simulink model "motor_control"  (R2021b)
settings: Solver=FixedStepAuto  StartTime=0.0  StopTime=inf  RelTol=1e-3  EnableMultiTasking=on
libraries: arduinomotorcarrierlib x4, simulink x2, arduinolib x1
settings Model: ExtModeTrigDuration=2  Creator=bkhusain  LastModifiedBy=cirie
settings SolverCC: AlgebraicLoopSolver=TrustRegion
settings OptimizationCC: EnhancedBackFolding=on  PassReuseOutputArgsAs=Individual arguments  ZeroExternalMemoryAtStartup=off  ZeroInternalMemoryAtStartup=off  MaxStackSize=64  OptimizeBlockOrder=speed  DifferentSizesBufferReuse=on  OptimizationCustomize=off  EfficientTunableParamExpr=on
settings DebuggingCC: ParameterTunabilityLossMsg=error  SFMachineParentedDataDiag=warning
settings HardwareCC: ProdBitPerPointer=32  ProdBitPerSizeT=32  ProdBitPerPtrDiffT=32  ProdLargestAtomicInteger=Long  ProdLargestAtomicFloat=Double  ProdWordSize=32  ProdHWDeviceType=ARM Compatible->ARM Cortex
settings SFSimCC: MATLABDynamicMemAlloc=off
settings RTWCC: Description=Embedded Coder  SystemTargetFile=ert.tlc  HardwareBoard=Arduino MKR WiFi 1010  TemplateMakefile=ert_default_tmf  Toolchain=Arduino ARM  BuildConfiguration=Faster Runs
settings CodeAppCC: ForceParamTrailComments=on  IgnoreCustomStorageClasses=off  OperatorAnnotations=on  SimulinkDataObjDesc=on  SFDataObjDesc=on  InsertBlockDesc=on
settings ERTTargetCC: SupportContinuousTime=on  SupportVariableSizeSignals=on  ExtModeTransport=3  ExtModeStaticAlloc=on  ExtModeStaticAllocSize=8192  ExtModeMexFile=ext_xcp  ExtModeIntrfLevel=Level2 - Open

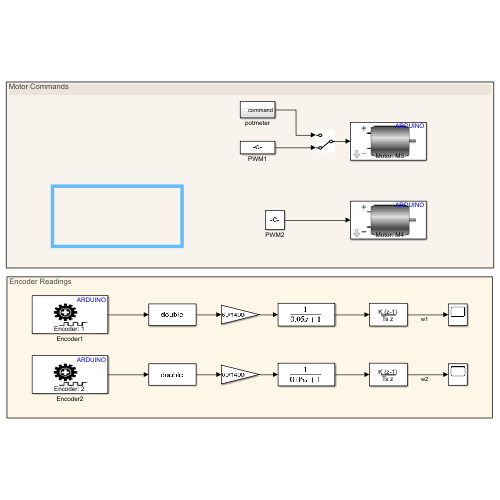
[thumbnail: Simulink's stored preview of the top-level diagram]
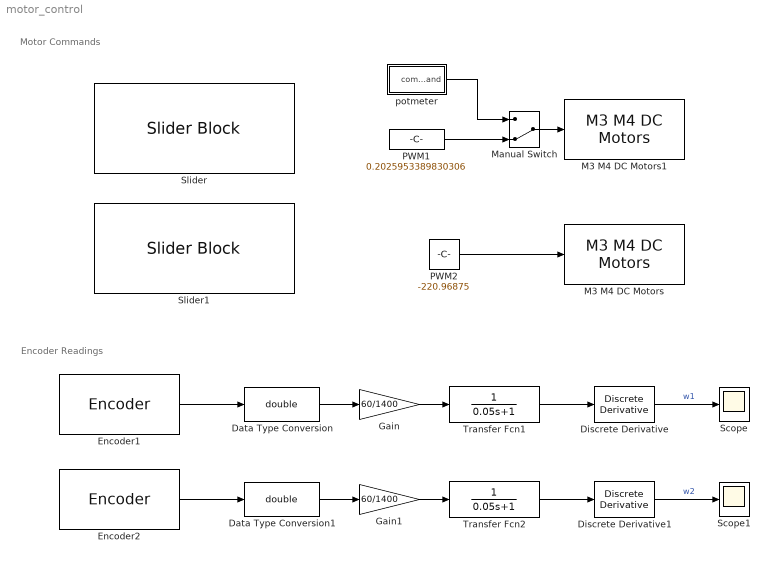
== system motor_control ==
  note: Encoder Readings
  note: Motor Commands
  Data Type Conversion : DataTypeConversion  OutDataTypeStr=double
  Data Type Conversion1 : DataTypeConversion  OutDataTypeStr=double
  Discrete Derivative : simulink/Discrete/Discrete Derivative  gainval=1.0  ICPrevScaledInput=0.0  OutMin=[]  OutMax=[]  OutDataType=fixdt(1, 16)  OutScaling=2^-10  DoSatur=off
  Discrete Derivative1 : simulink/Discrete/Discrete Derivative  gainval=1.0  ICPrevScaledInput=0.0  OutMin=[]  OutMax=[]  OutDataType=fixdt(1, 16)  OutScaling=2^-10  DoSatur=off
  Encoder1 : arduinomotorcarrierlib/Encoder  SlaveAddress=uint8( hex2dec( '66' ) )  blockPlatform=ARDUINO  Encoder=1  ShowSpeed=off  ResetOption=on  SampleTime=0.05
      settings: SourceProductBaseCode=ARDUINO
  Encoder2 : arduinomotorcarrierlib/Encoder  SlaveAddress=uint8( hex2dec( '66' ) )  blockPlatform=ARDUINO  Encoder=2  ShowSpeed=off  ResetOption=on  SampleTime=0.05
      settings: SourceProductBaseCode=ARDUINO
  Gain : Gain  Gain=60/1400
  Gain1 : Gain  Gain=60/1400
  M3 M4 DC Motors : arduinomotorcarrierlib/M3 M4 DC Motors  MotorNumber=M4  forwardPinNumber=4  reversePinNumber=5
      settings: SourceProductBaseCode=ARDUINO
  M3 M4 DC Motors1 : arduinomotorcarrierlib/M3 M4 DC Motors  MotorNumber=M3  forwardPinNumber=3  reversePinNumber=2
      settings: SourceProductBaseCode=ARDUINO
  Manual Switch : ManualSwitch  CurrentSetting=0
  PWM1 : Constant  Value=0.2025953389830306
  PWM2 : Constant  Value=-220.96875
  Scope : Scope
  Scope1 : Scope
  Slider : SliderBlock  ScaleMin=-255  ScaleMax=255
  Slider1 : SliderBlock  ScaleMin=-255  ScaleMax=255
  Transfer Fcn1 : TransferFcn  Denominator=[0.05 1]
  Transfer Fcn2 : TransferFcn  Denominator=[0.05 1]
  potmeter : Subsystem
  wires:
  PWM2/1 -> M3 M4 DC Motors/1
  Encoder1/1 -> Data Type Conversion/1
  Transfer Fcn1/1 -> Discrete Derivative/1
  Gain/1 -> Transfer Fcn1/1
  Data Type Conversion/1 -> Gain/1
  Discrete Derivative/1 -> Scope/1  "w1"
  PWM1/1 -> Manual Switch/2
  Discrete Derivative1/1 -> Scope1/1  "w2"
  Data Type Conversion1/1 -> Gain1/1
  Gain1/1 -> Transfer Fcn2/1
  Transfer Fcn2/1 -> Discrete Derivative1/1
  Encoder2/1 -> Data Type Conversion1/1
  Manual Switch/1 -> M3 M4 DC Motors1/1
  potmeter/1(command) -> Manual Switch/1

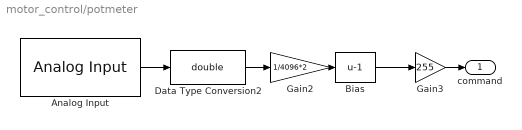
== system motor_control/potmeter ==
  Analog Input : arduinolib/Analog Input  pinNumber=5  ReadResultsOnly=off  ConversionTriggerSource=Software  ExternalTriggerType=uint32( 0 )  OutputDataType=uint16  EnableConversionCompleteNotify=off  EnableOuputStatus=off  SampleTime=-1  blockPlatform=arduino
  Bias : Bias  Bias=-1
  Data Type Conversion2 : DataTypeConversion  OutDataTypeStr=double
  Gain2 : Gain  Gain=1/4096*2
  Gain3 : Gain  Gain=255
  command : Outport
  wires:
  Bias/1 -> Gain3/1
  Data Type Conversion2/1 -> Gain2/1
  Analog Input/1 -> Data Type Conversion2/1
  Gain2/1 -> Bias/1
  Gain3/1 -> command/1
